simulink model "Ejercicio1"  (R2023b)
settings: Solver=VariableStepAuto  StartTime=0.0  StopTime=120  MaxStep=0.05  RelTol=1e-3
undefined symbols (not defined in the file): b, k, m, sys1
settings Model: Creator=lopez  LastModifiedBy=lopez

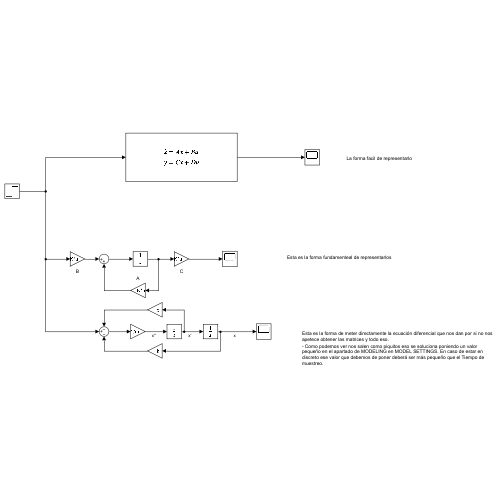
[thumbnail: Simulink's stored preview of the top-level diagram]
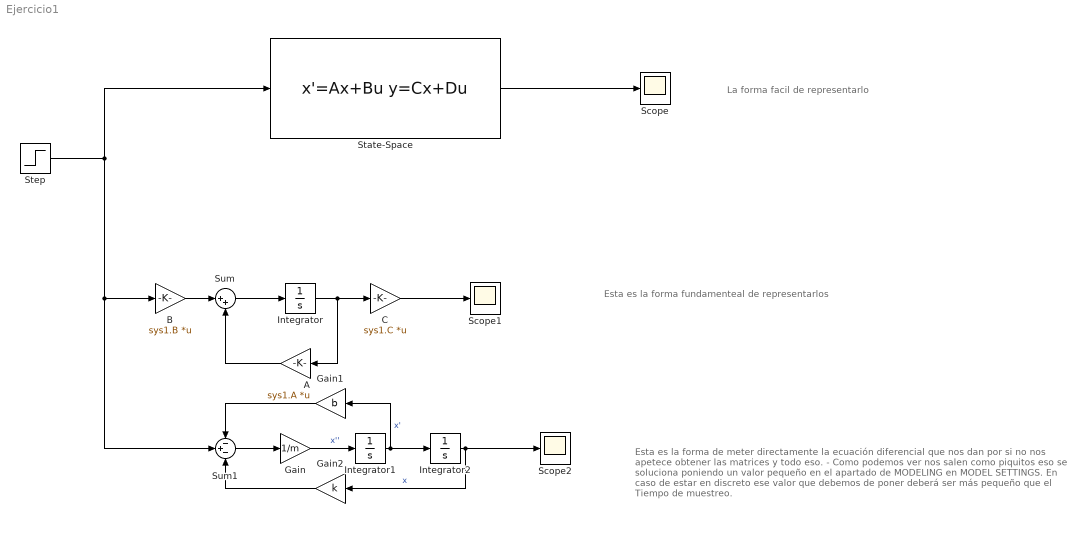
== system Ejercicio1 ==
  note: La forma facil de representarlo
  note: Esta es la forma fundamenteal de representarlos
  note: Esta es la forma de meter directamente la ecuación diferencial que nos dan por si no nos apetece obtener las matrices y todo eso.
      | - Como podemos ver nos salen como piquitos eso se soluciona poniendo un valor pequeño en el apartado de MODELING en MODEL SETTINGS. En caso de estar en discreto ese valor que debemos de poner deberá ser más pequeño que el Tiempo de muestreo.
  A : Gain  Gain=sys1.A  Multiplication=Matrix(K*u)
  B : Gain  Gain=sys1.B  Multiplication=Matrix(K*u)
  C : Gain  Gain=sys1.C  Multiplication=Matrix(K*u)
  Gain : Gain  Gain=1/m
  Gain1 : Gain  Gain=b
  Gain2 : Gain  Gain=k
  Integrator : Integrator
  Integrator1 : Integrator
  Integrator2 : Integrator
  Scope : Scope
  Scope1 : Scope
  Scope2 : Scope
  State-Space : StateSpace  A=sys1.A  B=sys1.B  C=sys1.C  D=sys1.D  InitialCondition=0
  Step : Step  SampleTime=0
  Sum : Sum  Inputs=|++
  Sum1 : Sum  Inputs=-+-
  wires:
  Step/1 -> Sum1/2, B/1, State-Space/1
  State-Space/1 -> Scope/1
  A/1 -> Sum/2
  C/1 -> Scope1/1
  Sum/1 -> Integrator/1
  Integrator/1 -> A/1, C/1
  B/1 -> Sum/1
  Sum1/1 -> Gain/1
  Gain/1 -> Integrator1/1  "x''"
  Integrator1/1 -> Gain1/1, Integrator2/1  "x'"
  Integrator2/1 -> Gain2/1, Scope2/1  "x"
  Gain1/1 -> Sum1/1
  Gain2/1 -> Sum1/3
